simulink library "halin"  (R2021b)
settings: Solver=VariableStepAuto  StartTime=0.0  StopTime=10.0  RelTol=1e-3
undefined symbols (not defined in the file): KHAL_CAN1ABM1E2E_flg, KHAL_CAN1EPB1E2E_flg, KHAL_CAN1EPS1E2E_flg, KHAL_CAN1ESC1E2E_flg, KHAL_CAN1ESC5E2E_flg, KHAL_CAN3BMS1E2E_flg, KHAL_CAN3BMS6E2E_flg, KHAL_CAN3CCU1E2E_flg, KHAL_CAN3CCU2E2E_flg, KHAL_CAN3MCUNF1E2E_flg, KHAL_CAN3MCUNR1E2E_flg, KHAL_CAN3Shifter1E2E_flg, KHAL_CAN3Shifter2E2E_flg, KHAL_CAN6FCM2E2E_flg, KHAL_CAN6FCM4E2E_flg, TRUE
libraries: simulink x645, FVT_lib x212, hcu_lib x59
(part 10 of 23)

== system halin/HAL_IN/CAN2/VHAL_CANMsgInvalidMETER1_flg ==
  Cast To Boolean13 : DataTypeConversion  OutDataTypeStr=boolean
  Constant : Constant  Value=TRUE
  Latch13 : hcu_lib/Basic_Blocks/Latch
  Switch13 : Switch  Criteria=u2 ~= 0
  Unit Delay : UnitDelay  SampleTime=-1  HasFrameUpgradeWarning=on
  UnitConverter : DataTypeConversion  OutDataTypeStr=boolean
  Out : Outport
  wires:
  Constant/1 -> Switch13/3
  Unit Delay/1 -> Cast To Boolean13/1
  Cast To Boolean13/1 -> Switch13/1, Latch13/1
  Switch13/1 -> UnitConverter/1
  Latch13/1 -> Switch13/2
  UnitConverter/1 -> Unit Delay/1, Out/1  "VHAL_CANMsgInvalidMETER1_flg"

== system halin/HAL_IN/CAN3/BMS1 ==
  DT_CAN3_SG_BMS1 : Inport
  0x3C : Constant  Value=0x3C
  0xDC : Constant  Value=0xDC
  BMSChckSum1 : Subsystem
  BMSRolCnct1 : Subsystem
  BitwiseAND{,1..17} (18 alike) : simulink/Logic and Bit Operations/Bitwise Operator  logicop=AND  UseBitMask=on  BitMask=0xFF  BitMaskRealWorld=Stored Integer
  BitwiseOR{,1..6,8..9,11..12,14} (12 alike) : simulink/Logic and Bit Operations/Bitwise Operator  logicop=OR  UseBitMask=off  BitMask=bin2dec('11011001')  BitMaskRealWorld=Stored Integer
  BitwiseOR10 : simulink/Logic and Bit Operations/Bitwise Operator  logicop=OR  UseBitMask=off  NumInputPorts=2  BitMask=bin2dec('11011001')  BitMaskRealWorld=Stored Integer
  BitwiseOR13 : simulink/Logic and Bit Operations/Bitwise Operator  logicop=OR  UseBitMask=off  NumInputPorts=2  BitMask=bin2dec('11011001')  BitMaskRealWorld=Stored Integer
  BitwiseOR7 : simulink/Logic and Bit Operations/Bitwise Operator  logicop=OR  UseBitMask=off  NumInputPorts=2  BitMask=bin2dec('11011001')  BitMaskRealWorld=Stored Integer
  DDM_CS&RC_Comparison : FVT_lib/hal/DDM_CS&RC_Comparison  MsgCycleTime=10
  Data Type Conversion{,1..17} (18 alike) : DataTypeConversion  OutDataTypeStr=uint8
  HVBPwrAvailChrg : Subsystem
  HVBPwrAvailChrg30 : Subsystem
  HVBPwrAvailChrg60 : Subsystem
  HVBPwrAvailDchrg : Subsystem
  HVBPwrAvailDchrg30 : Subsystem
  HVBPwrAvailDchrg60 : Subsystem
  HVBattCurr : Subsystem
  HVBattVolt : Subsystem
  KHAL_CAN3BMS1E2E_flg : Constant  Value=KHAL_CAN3BMS1E2E_flg
  LeftShift : ArithShift  BitShiftDirection=Left
  LeftShift1 : ArithShift  BitShiftDirection=Left
  MessageRollingCounter : FVT_lib/hal/MessageRollingCounter  CounterMAX=14  task_time_ms=5  msg_time_ms=10
  Mux : Mux  Inputs=15
  RightShift{,2,4,12,14} (5 alike) : ArithShift  BitShiftNumber=8
  RightShift{1,3,5,13,15} (5 alike) : ArithShift
  RightShift10 : ArithShift  BitShiftNumber=4
  RightShift11 : ArithShift  BitShiftNumber=-4
  RightShift6 : ArithShift  BitShiftNumber=4
  RightShift7 : ArithShift  BitShiftNumber=-4
  RightShift8 : ArithShift  BitShiftNumber=4
  RightShift9 : ArithShift  BitShiftNumber=-4
  bus_selector : BusSelector  OutputSignals=CAN3_BMSChckSum_1,CAN3_BMSRolCnct_1,CAN3_HVBPwrAvailChrg,CAN3_HVBPwrAvailChrg30,CAN3_HVBPwrAvailChrg60,CAN3_HVBPwrAvailDchrg,CAN3_HVBPwrAvailDchrg30,CAN3_HVBPwrAvailDchrg60,CAN3_HVBattCurr,CAN3_HVBattVolt
  bus_selector1 : BusSelector  OutputSignals=CAN3_BMSChckSum_1
  bus_selector10 : BusSelector  OutputSignals=CAN3_HVBattVolt
  bus_selector2 : BusSelector  OutputSignals=CAN3_BMSRolCnct_1
  bus_selector3 : BusSelector  OutputSignals=CAN3_HVBPwrAvailChrg
  bus_selector4 : BusSelector  OutputSignals=CAN3_HVBPwrAvailChrg30
  bus_selector5 : BusSelector  OutputSignals=CAN3_HVBPwrAvailChrg60
  bus_selector6 : BusSelector  OutputSignals=CAN3_HVBPwrAvailDchrg
  bus_selector7 : BusSelector  OutputSignals=CAN3_HVBPwrAvailDchrg30
  bus_selector8 : BusSelector  OutputSignals=CAN3_HVBPwrAvailDchrg60
  bus_selector9 : BusSelector  OutputSignals=CAN3_HVBattCurr
  constant : Constant  Value=0x0  OutDataTypeStr=uint8
  VHAL_BMS1CSErr_flg : Outport
  VHAL_BMS1RCErr_flg : Outport  Port=2
  VHAL_BMSChckSum1_enum : Outport  Port=3
  VHAL_BMSRolCnct1_enum : Outport  Port=4
  VHAL_HVBPwrAvailChrg_kW : Outport  Port=5
  VHAL_HVBPwrAvailChrg30_kW : Outport  Port=6
  VHAL_HVBPwrAvailChrg60_kW : Outport  Port=7
  VHAL_HVBPwrAvailDchrg_kW : Outport  Port=8
  VHAL_HVBPwrAvailDchrg30_kW : Outport  Port=9
  VHAL_HVBPwrAvailDchrg60_kW : Outport  Port=10
  VHAL_HVBattCurr_A : Outport  Port=11
  VHAL_HVBattVolt_V : Outport  Port=12
  wires:
  DT_CAN3_SG_BMS1/1 -> [DT_CAN3_SG_BMS1]
  [DT_CAN3_SG_BMS1] -> bus_selector/1
  bus_selector/1 -> [CAN3_BMSChckSum_1]  "<CAN3_BMSChckSum_1>"
  [CAN3_BMSChckSum_1] -> LeftShift/1
  LeftShift/1 -> BitwiseAND/1
  BitwiseAND/1 -> [Byte_0_CAN3_BMSChckSum_1]
  bus_selector/2 -> [CAN3_BMSRolCnct_1]  "<CAN3_BMSRolCnct_1>"
  [CAN3_BMSRolCnct_1] -> LeftShift1/1
  LeftShift1/1 -> BitwiseAND1/1
  BitwiseAND1/1 -> [Byte_1_CAN3_BMSRolCnct_1]
  bus_selector/3 -> [CAN3_HVBPwrAvailChrg]  "<CAN3_HVBPwrAvailChrg>"
  [CAN3_HVBPwrAvailChrg] -> RightShift/1, RightShift1/1
  RightShift/1 -> BitwiseAND2/1
  BitwiseAND2/1 -> [Byte_11_CAN3_HVBPwrAvailChrg]
  RightShift1/1 -> BitwiseAND3/1
  BitwiseAND3/1 -> [Byte_12_CAN3_HVBPwrAvailChrg]
  bus_selector/4 -> [CAN3_HVBPwrAvailChrg30]  "<CAN3_HVBPwrAvailChrg30>"
  [CAN3_HVBPwrAvailChrg30] -> RightShift2/1, RightShift3/1
  RightShift2/1 -> BitwiseAND4/1
  BitwiseAND4/1 -> [Byte_14_CAN3_HVBPwrAvailChrg30]
  RightShift3/1 -> BitwiseAND5/1
  BitwiseAND5/1 -> [Byte_15_CAN3_HVBPwrAvailChrg30]
  bus_selector/5 -> [CAN3_HVBPwrAvailChrg60]  "<CAN3_HVBPwrAvailChrg60>"
  [CAN3_HVBPwrAvailChrg60] -> RightShift4/1, RightShift5/1
  RightShift4/1 -> BitwiseAND6/1
  BitwiseAND6/1 -> [Byte_8_CAN3_HVBPwrAvailChrg60]
  RightShift5/1 -> BitwiseAND7/1
  BitwiseAND7/1 -> [Byte_9_CAN3_HVBPwrAvailChrg60]
  bus_selector/6 -> [CAN3_HVBPwrAvailDchrg]  "<CAN3_HVBPwrAvailDchrg>"
  [CAN3_HVBPwrAvailDchrg] -> RightShift6/1, RightShift7/1
  RightShift6/1 -> BitwiseAND8/1
  BitwiseAND8/1 -> [Byte_10_CAN3_HVBPwrAvailDchrg]
  RightShift7/1 -> BitwiseAND9/1
  BitwiseAND9/1 -> [Byte_11_CAN3_HVBPwrAvailDchrg]
  bus_selector/7 -> [CAN3_HVBPwrAvailDchrg30]  "<CAN3_HVBPwrAvailDchrg30>"
  [CAN3_HVBPwrAvailDchrg30] -> RightShift8/1, RightShift9/1
  RightShift8/1 -> BitwiseAND10/1
  BitwiseAND10/1 -> [Byte_13_CAN3_HVBPwrAvailDchrg30]
  RightShift9/1 -> BitwiseAND11/1
  BitwiseAND11/1 -> [Byte_14_CAN3_HVBPwrAvailDchrg30]
  bus_selector/8 -> [CAN3_HVBPwrAvailDchrg60]  "<CAN3_HVBPwrAvailDchrg60>"
  [CAN3_HVBPwrAvailDchrg60] -> RightShift10/1, RightShift11/1
  RightShift10/1 -> BitwiseAND12/1
  BitwiseAND12/1 -> [Byte_7_CAN3_HVBPwrAvailDchrg60]
  RightShift11/1 -> BitwiseAND13/1
  BitwiseAND13/1 -> [Byte_8_CAN3_HVBPwrAvailDchrg60]
  bus_selector/9 -> [CAN3_HVBattCurr]  "<CAN3_HVBattCurr>"
  [CAN3_HVBattCurr] -> RightShift12/1, RightShift13/1
  RightShift12/1 -> BitwiseAND14/1
  BitwiseAND14/1 -> [Byte_5_CAN3_HVBattCurr]
  RightShift13/1 -> BitwiseAND15/1
  BitwiseAND15/1 -> [Byte_6_CAN3_HVBattCurr]
  bus_selector/10 -> [CAN3_HVBattVolt]  "<CAN3_HVBattVolt>"
  [CAN3_HVBattVolt] -> RightShift14/1, RightShift15/1
  RightShift14/1 -> BitwiseAND16/1
  BitwiseAND16/1 -> [Byte_3_CAN3_HVBattVolt]
  RightShift15/1 -> BitwiseAND17/1
  BitwiseAND17/1 -> [Byte_4_CAN3_HVBattVolt]
  Data Type Conversion/1 -> BitwiseOR/1
  [Byte_0_CAN3_BMSChckSum_1] -> Data Type Conversion/1
  BitwiseOR/1 -> [Byte_0]
  Data Type Conversion1/1 -> BitwiseOR1/1
  [Byte_1_CAN3_BMSRolCnct_1] -> Data Type Conversion1/1
  BitwiseOR1/1 -> [Byte_1]
  constant/1 -> [Byte_2]
  Data Type Conversion2/1 -> BitwiseOR2/1
  [Byte_3_CAN3_HVBattVolt] -> Data Type Conversion2/1
  BitwiseOR2/1 -> [Byte_3]
  Data Type Conversion3/1 -> BitwiseOR3/1
  [Byte_4_CAN3_HVBattVolt] -> Data Type Conversion3/1
  BitwiseOR3/1 -> [Byte_4]
  Data Type Conversion4/1 -> BitwiseOR4/1
  [Byte_5_CAN3_HVBattCurr] -> Data Type Conversion4/1
  BitwiseOR4/1 -> [Byte_5]
  Data Type Conversion5/1 -> BitwiseOR5/1
  [Byte_6_CAN3_HVBattCurr] -> Data Type Conversion5/1
  BitwiseOR5/1 -> [Byte_6]
  Data Type Conversion6/1 -> BitwiseOR6/1
  [Byte_7_CAN3_HVBPwrAvailDchrg60] -> Data Type Conversion6/1
  BitwiseOR6/1 -> [Byte_7]
  Data Type Conversion7/1 -> BitwiseOR7/1
  [Byte_8_CAN3_HVBPwrAvailChrg60] -> Data Type Conversion7/1
  Data Type Conversion8/1 -> BitwiseOR7/2
  [Byte_8_CAN3_HVBPwrAvailDchrg60] -> Data Type Conversion8/1
  BitwiseOR7/1 -> [Byte_8]
  Data Type Conversion9/1 -> BitwiseOR8/1
  [Byte_9_CAN3_HVBPwrAvailChrg60] -> Data Type Conversion9/1
  BitwiseOR8/1 -> [Byte_9]
  Data Type Conversion10/1 -> BitwiseOR9/1
  [Byte_10_CAN3_HVBPwrAvailDchrg] -> Data Type Conversion10/1
  BitwiseOR9/1 -> [Byte_10]
  Data Type Conversion11/1 -> BitwiseOR10/1
  [Byte_11_CAN3_HVBPwrAvailChrg] -> Data Type Conversion11/1
  Data Type Conversion12/1 -> BitwiseOR10/2
  [Byte_11_CAN3_HVBPwrAvailDchrg] -> Data Type Conversion12/1
  BitwiseOR10/1 -> [Byte_11]
  Data Type Conversion13/1 -> BitwiseOR11/1
  [Byte_12_CAN3_HVBPwrAvailChrg] -> Data Type Conversion13/1
  BitwiseOR11/1 -> [Byte_12]
  Data Type Conversion14/1 -> BitwiseOR12/1
  [Byte_13_CAN3_HVBPwrAvailDchrg30] -> Data Type Conversion14/1
  BitwiseOR12/1 -> [Byte_13]
  Data Type Conversion15/1 -> BitwiseOR13/1
  [Byte_14_CAN3_HVBPwrAvailChrg30] -> Data Type Conversion15/1
  Data Type Conversion16/1 -> BitwiseOR13/2
  [Byte_14_CAN3_HVBPwrAvailDchrg30] -> Data Type Conversion16/1
  BitwiseOR13/1 -> [Byte_14]
  Data Type Conversion17/1 -> BitwiseOR14/1
  [Byte_15_CAN3_HVBPwrAvailChrg30] -> Data Type Conversion17/1
  BitwiseOR14/1 -> [Byte_15]
  [Byte_1] -> Mux/1
  [Byte_2] -> Mux/2
  [Byte_3] -> Mux/3
  [Byte_4] -> Mux/4
  [Byte_5] -> Mux/5
  [Byte_6] -> Mux/6
  [Byte_7] -> Mux/7
  [Byte_8] -> Mux/8
  [Byte_9] -> Mux/9
  [Byte_10] -> Mux/10
  [Byte_11] -> Mux/11
  [Byte_12] -> Mux/12
  [Byte_13] -> Mux/13
  [Byte_14] -> Mux/14
  [Byte_15] -> Mux/15
  Mux/1 -> [VHAL_CAN3BMS1noCS_raw]
  KHAL_CAN3BMS1E2E_flg/1 -> DDM_CS&RC_Comparison/1
  0x3C/1 -> DDM_CS&RC_Comparison/2
  0xDC/1 -> DDM_CS&RC_Comparison/3
  [VHAL_CAN3BMS1noCS_raw] -> DDM_CS&RC_Comparison/4
  [Byte_0] -> DDM_CS&RC_Comparison/5
  [RC_ECU] -> DDM_CS&RC_Comparison/6
  MessageRollingCounter/1 -> DDM_CS&RC_Comparison/7
  DDM_CS&RC_Comparison/1 -> VHAL_BMS1CSErr_flg/1
  DDM_CS&RC_Comparison/2 -> VHAL_BMS1RCErr_flg/1
  [DT_CAN3_SG_BMS1] -> bus_selector1/1
  bus_selector1/1 -> BMSChckSum1/1(BMSChckSum_1)  "<CAN3_BMSChckSum_1>"
  BMSChckSum1/1(VHAL_BMSChckSum1_enum) -> VHAL_BMSChckSum1_enum/1
  [DT_CAN3_SG_BMS1] -> bus_selector2/1
  bus_selector2/1 -> BMSRolCnct1/1(BMSRolCnct_1)  "<CAN3_BMSRolCnct_1>"
  BMSRolCnct1/1(VHAL_BMSRolCnct1_enum) -> VHAL_BMSRolCnct1_enum/1, [RC_ECU]
  [DT_CAN3_SG_BMS1] -> bus_selector3/1
  bus_selector3/1 -> HVBPwrAvailChrg/1(HVBPwrAvailChrg)  "<CAN3_HVBPwrAvailChrg>"
  HVBPwrAvailChrg/1(VHAL_HVBPwrAvailChrg_kW) -> VHAL_HVBPwrAvailChrg_kW/1
  [DT_CAN3_SG_BMS1] -> bus_selector4/1
  bus_selector4/1 -> HVBPwrAvailChrg30/1(HVBPwrAvailChrg30)  "<CAN3_HVBPwrAvailChrg30>"
  HVBPwrAvailChrg30/1(VHAL_HVBPwrAvailChrg30_kW) -> VHAL_HVBPwrAvailChrg30_kW/1
  [DT_CAN3_SG_BMS1] -> bus_selector5/1
  bus_selector5/1 -> HVBPwrAvailChrg60/1(HVBPwrAvailChrg60)  "<CAN3_HVBPwrAvailChrg60>"
  HVBPwrAvailChrg60/1(VHAL_HVBPwrAvailChrg60_kW) -> VHAL_HVBPwrAvailChrg60_kW/1
  [DT_CAN3_SG_BMS1] -> bus_selector6/1
  bus_selector6/1 -> HVBPwrAvailDchrg/1(HVBPwrAvailDchrg)  "<CAN3_HVBPwrAvailDchrg>"
  HVBPwrAvailDchrg/1(VHAL_HVBPwrAvailDchrg_kW) -> VHAL_HVBPwrAvailDchrg_kW/1
  [DT_CAN3_SG_BMS1] -> bus_selector7/1
  bus_selector7/1 -> HVBPwrAvailDchrg30/1(HVBPwrAvailDchrg30)  "<CAN3_HVBPwrAvailDchrg30>"
  HVBPwrAvailDchrg30/1(VHAL_HVBPwrAvailDchrg30_kW) -> VHAL_HVBPwrAvailDchrg30_kW/1
  [DT_CAN3_SG_BMS1] -> bus_selector8/1
  bus_selector8/1 -> HVBPwrAvailDchrg60/1(HVBPwrAvailDchrg60)  "<CAN3_HVBPwrAvailDchrg60>"
  HVBPwrAvailDchrg60/1(VHAL_HVBPwrAvailDchrg60_kW) -> VHAL_HVBPwrAvailDchrg60_kW/1
  [DT_CAN3_SG_BMS1] -> bus_selector9/1
  bus_selector9/1 -> HVBattCurr/1(HVBattCurr)  "<CAN3_HVBattCurr>"
  HVBattCurr/1(VHAL_HVBattCurr_A) -> VHAL_HVBattCurr_A/1
  [DT_CAN3_SG_BMS1] -> bus_selector10/1
  bus_selector10/1 -> HVBattVolt/1(HVBattVolt)  "<CAN3_HVBattVolt>"
  HVBattVolt/1(VHAL_HVBattVolt_V) -> VHAL_HVBattVolt_V/1

== system halin/HAL_IN/CAN3/BMS3 ==
  DT_CAN3_SG_BMS3 : Inport
  ACChrgCurrDis : Subsystem
  FireDetErr : Subsystem
  HVBChrgPwr : Subsystem
  HVBChrgPwrTotal : Subsystem
  HVBDrvPwr : Subsystem
  HVBDrvPwrTotal : Subsystem
  HVBFullChrgPwr : Subsystem
  HVBIsoImpedenceN : Subsystem
  HVBIsoImpedenceP : Subsystem
  HVBSOH : Subsystem
  HVBattErr : Subsystem
  HVBattPackVolt : Subsystem
  HVBattSOC : Subsystem
  HVBattSOCDis : Subsystem
  RemainChrgTime : Subsystem
  bus_selector : BusSelector  OutputSignals=CAN3_ACChrgCurrDis
  bus_selector1 : BusSelector  OutputSignals=CAN3_FireDetErr
  bus_selector10 : BusSelector  OutputSignals=CAN3_HVBattErr
  bus_selector11 : BusSelector  OutputSignals=CAN3_HVBattPackVolt
  bus_selector12 : BusSelector  OutputSignals=CAN3_HVBattSOC
  bus_selector13 : BusSelector  OutputSignals=CAN3_HVBattSOCDis
  bus_selector14 : BusSelector  OutputSignals=CAN3_RemainChrgTime
  bus_selector2 : BusSelector  OutputSignals=CAN3_HVBChrgPwr
  bus_selector3 : BusSelector  OutputSignals=CAN3_HVBChrgPwrTotal
  bus_selector4 : BusSelector  OutputSignals=CAN3_HVBDrvPwr
  bus_selector5 : BusSelector  OutputSignals=CAN3_HVBDrvPwrTotal
  bus_selector6 : BusSelector  OutputSignals=CAN3_HVBFullChrgPwr
  bus_selector7 : BusSelector  OutputSignals=CAN3_HVBIsoImpedenceN
  bus_selector8 : BusSelector  OutputSignals=CAN3_HVBIsoImpedenceP
  bus_selector9 : BusSelector  OutputSignals=CAN3_HVBSOH
  VHAL_ACChrgCurrDis_A : Outport
  VHAL_FireDetErr_flg : Outport  Port=2
  VHAL_HVBChrgPwr_kWh : Outport  Port=3
  VHAL_HVBChrgPwrTotal_kWh : Outport  Port=4
  VHAL_HVBDrvPwr_kWh : Outport  Port=5
  VHAL_HVBDrvPwrTotal_kWh : Outport  Port=6
  VHAL_HVBFullChrgPwr_kWh : Outport  Port=7
  VHAL_HVBIsoImpedenceN_Megaohm : Outport  Port=8
  VHAL_HVBIsoImpedenceP_Megaohm : Outport  Port=9
  VHAL_HVBSOH_pct : Outport  Port=10
  VHAL_HVBattErr_flg : Outport  Port=11
  VHAL_HVBattPackVolt_V : Outport  Port=12
  VHAL_HVBattSOC_pct : Outport  Port=13
  VHAL_HVBattSOCDis_pct : Outport  Port=14
  VHAL_RemainChrgTime_min : Outport  Port=15
  wires:
  DT_CAN3_SG_BMS3/1 -> [DT_CAN3_SG_BMS3]
  [DT_CAN3_SG_BMS3] -> bus_selector/1
  bus_selector/1 -> ACChrgCurrDis/1(ACChrgCurrDis)  "<CAN3_ACChrgCurrDis>"
  ACChrgCurrDis/1(VHAL_ACChrgCurrDis_A) -> VHAL_ACChrgCurrDis_A/1
  [DT_CAN3_SG_BMS3] -> bus_selector1/1
  bus_selector1/1 -> FireDetErr/1(FireDetErr)  "<CAN3_FireDetErr>"
  FireDetErr/1(VHAL_FireDetErr_flg) -> VHAL_FireDetErr_flg/1
  [DT_CAN3_SG_BMS3] -> bus_selector2/1
  bus_selector2/1 -> HVBChrgPwr/1(HVBChrgPwr)  "<CAN3_HVBChrgPwr>"
  HVBChrgPwr/1(VHAL_HVBChrgPwr_kWh) -> VHAL_HVBChrgPwr_kWh/1
  [DT_CAN3_SG_BMS3] -> bus_selector3/1
  bus_selector3/1 -> HVBChrgPwrTotal/1(HVBChrgPwrTotal)  "<CAN3_HVBChrgPwrTotal>"
  HVBChrgPwrTotal/1(VHAL_HVBChrgPwrTotal_kWh) -> VHAL_HVBChrgPwrTotal_kWh/1
  [DT_CAN3_SG_BMS3] -> bus_selector4/1
  bus_selector4/1 -> HVBDrvPwr/1(HVBDrvPwr)  "<CAN3_HVBDrvPwr>"
  HVBDrvPwr/1(VHAL_HVBDrvPwr_kWh) -> VHAL_HVBDrvPwr_kWh/1
  [DT_CAN3_SG_BMS3] -> bus_selector5/1
  bus_selector5/1 -> HVBDrvPwrTotal/1(HVBDrvPwrTotal)  "<CAN3_HVBDrvPwrTotal>"
  HVBDrvPwrTotal/1(VHAL_HVBDrvPwrTotal_kWh) -> VHAL_HVBDrvPwrTotal_kWh/1
  [DT_CAN3_SG_BMS3] -> bus_selector6/1
  bus_selector6/1 -> HVBFullChrgPwr/1(HVBFullChrgPwr)  "<CAN3_HVBFullChrgPwr>"
  HVBFullChrgPwr/1(VHAL_HVBFullChrgPwr_kWh) -> VHAL_HVBFullChrgPwr_kWh/1
  [DT_CAN3_SG_BMS3] -> bus_selector7/1
  bus_selector7/1 -> HVBIsoImpedenceN/1(HVBIsoImpedenceN)  "<CAN3_HVBIsoImpedenceN>"
  HVBIsoImpedenceN/1(VHAL_HVBIsoImpedenceN_Megaohm) -> VHAL_HVBIsoImpedenceN_Megaohm/1
  [DT_CAN3_SG_BMS3] -> bus_selector8/1
  bus_selector8/1 -> HVBIsoImpedenceP/1(HVBIsoImpedenceP)  "<CAN3_HVBIsoImpedenceP>"
  HVBIsoImpedenceP/1(VHAL_HVBIsoImpedenceP_Megaohm) -> VHAL_HVBIsoImpedenceP_Megaohm/1
  [DT_CAN3_SG_BMS3] -> bus_selector9/1
  bus_selector9/1 -> HVBSOH/1(HVBSOH)  "<CAN3_HVBSOH>"
  HVBSOH/1(VHAL_HVBSOH_pct) -> VHAL_HVBSOH_pct/1
  [DT_CAN3_SG_BMS3] -> bus_selector10/1
  bus_selector10/1 -> HVBattErr/1(HVBattErr)  "<CAN3_HVBattErr>"
  HVBattErr/1(VHAL_HVBattErr_flg) -> VHAL_HVBattErr_flg/1
  [DT_CAN3_SG_BMS3] -> bus_selector11/1
  bus_selector11/1 -> HVBattPackVolt/1(HVBattPackVolt)  "<CAN3_HVBattPackVolt>"
  HVBattPackVolt/1(VHAL_HVBattPackVolt_V) -> VHAL_HVBattPackVolt_V/1
  [DT_CAN3_SG_BMS3] -> bus_selector12/1
  bus_selector12/1 -> HVBattSOC/1(HVBattSOC)  "<CAN3_HVBattSOC>"
  HVBattSOC/1(VHAL_HVBattSOC_pct) -> VHAL_HVBattSOC_pct/1
  [DT_CAN3_SG_BMS3] -> bus_selector13/1
  bus_selector13/1 -> HVBattSOCDis/1(HVBattSOCDis)  "<CAN3_HVBattSOCDis>"
  HVBattSOCDis/1(VHAL_HVBattSOCDis_pct) -> VHAL_HVBattSOCDis_pct/1
  [DT_CAN3_SG_BMS3] -> bus_selector14/1
  bus_selector14/1 -> RemainChrgTime/1(RemainChrgTime)  "<CAN3_RemainChrgTime>"
  RemainChrgTime/1(VHAL_RemainChrgTime_min) -> VHAL_RemainChrgTime_min/1

== system halin/HAL_IN/CAN3/BMS4 ==
  DT_CAN3_SG_BMS4 : Inport
  CellTempAvg : Subsystem
  HVBCellVoltMax : Subsystem
  HVBCellVoltMin : Subsystem
  HVBMTempMax : Subsystem
  HVBMTempMin : Subsystem
  MaxCellTempNum : Subsystem
  MaxCellVoltNum : Subsystem
  MinCellTempNum : Subsystem
  MinCellVoltNum : Subsystem
  bus_selector : BusSelector  OutputSignals=CAN3_CellTempAvg
  bus_selector1 : BusSelector  OutputSignals=CAN3_HVBCellVoltMax
  bus_selector2 : BusSelector  OutputSignals=CAN3_HVBCellVoltMin
  bus_selector3 : BusSelector  OutputSignals=CAN3_HVBMTempMax
  bus_selector4 : BusSelector  OutputSignals=CAN3_HVBMTempMin
  bus_selector5 : BusSelector  OutputSignals=CAN3_MaxCellTemp_Num
  bus_selector6 : BusSelector  OutputSignals=CAN3_MaxCellVolt_Num
  bus_selector7 : BusSelector  OutputSignals=CAN3_MinCellTemp_Num
  bus_selector8 : BusSelector  OutputSignals=CAN3_MinCellVolt_Num
  VHAL_CellTempAvg_C : Outport
  VHAL_HVBCellVoltMax_mV : Outport  Port=2
  VHAL_HVBCellVoltMin_mV : Outport  Port=3
  VHAL_HVBMTempMax_C : Outport  Port=4
  VHAL_HVBMTempMin_C : Outport  Port=5
  VHAL_MaxCellTempNum_enum : Outport  Port=6
  VHAL_MaxCellVoltNum_enum : Outport  Port=7
  VHAL_MinCellTempNum_enum : Outport  Port=8
  VHAL_MinCellVoltNum_enum : Outport  Port=9
  wires:
  DT_CAN3_SG_BMS4/1 -> [DT_CAN3_SG_BMS4]
  [DT_CAN3_SG_BMS4] -> bus_selector/1
  bus_selector/1 -> CellTempAvg/1(CellTempAvg)  "<CAN3_CellTempAvg>"
  CellTempAvg/1(VHAL_CellTempAvg_C) -> VHAL_CellTempAvg_C/1
  [DT_CAN3_SG_BMS4] -> bus_selector1/1
  bus_selector1/1 -> HVBCellVoltMax/1(HVBCellVoltMax)  "<CAN3_HVBCellVoltMax>"
  HVBCellVoltMax/1(VHAL_HVBCellVoltMax_mV) -> VHAL_HVBCellVoltMax_mV/1
  [DT_CAN3_SG_BMS4] -> bus_selector2/1
  bus_selector2/1 -> HVBCellVoltMin/1(HVBCellVoltMin)  "<CAN3_HVBCellVoltMin>"
  HVBCellVoltMin/1(VHAL_HVBCellVoltMin_mV) -> VHAL_HVBCellVoltMin_mV/1
  [DT_CAN3_SG_BMS4] -> bus_selector3/1
  bus_selector3/1 -> HVBMTempMax/1(HVBMTempMax)  "<CAN3_HVBMTempMax>"
  HVBMTempMax/1(VHAL_HVBMTempMax_C) -> VHAL_HVBMTempMax_C/1
  [DT_CAN3_SG_BMS4] -> bus_selector4/1
  bus_selector4/1 -> HVBMTempMin/1(HVBMTempMin)  "<CAN3_HVBMTempMin>"
  HVBMTempMin/1(VHAL_HVBMTempMin_C) -> VHAL_HVBMTempMin_C/1
  [DT_CAN3_SG_BMS4] -> bus_selector5/1
  bus_selector5/1 -> MaxCellTempNum/1(MaxCellTemp_Num)  "<CAN3_MaxCellTemp_Num>"
  MaxCellTempNum/1(VHAL_MaxCellTempNum_enum) -> VHAL_MaxCellTempNum_enum/1
  [DT_CAN3_SG_BMS4] -> bus_selector6/1
  bus_selector6/1 -> MaxCellVoltNum/1(MaxCellVolt_Num)  "<CAN3_MaxCellVolt_Num>"
  MaxCellVoltNum/1(VHAL_MaxCellVoltNum_enum) -> VHAL_MaxCellVoltNum_enum/1
  [DT_CAN3_SG_BMS4] -> bus_selector7/1
  bus_selector7/1 -> MinCellTempNum/1(MinCellTemp_Num)  "<CAN3_MinCellTemp_Num>"
  MinCellTempNum/1(VHAL_MinCellTempNum_enum) -> VHAL_MinCellTempNum_enum/1
  [DT_CAN3_SG_BMS4] -> bus_selector8/1
  bus_selector8/1 -> MinCellVoltNum/1(MinCellVolt_Num)  "<CAN3_MinCellVolt_Num>"
  MinCellVoltNum/1(VHAL_MinCellVoltNum_enum) -> VHAL_MinCellVoltNum_enum/1

== system halin/HAL_IN/CAN3/BMS5 ==
  DT_CAN3_SG_BMS5 : Inport
  HVInVolt : Subsystem
  LVBattDet12V : Subsystem
  OBCACCSLimit : Subsystem
  OBCDCCurLm : Subsystem
  OBCDCVoltLm : Subsystem
  bus_selector : BusSelector  OutputSignals=CAN3_HVInVolt
  bus_selector1 : BusSelector  OutputSignals=CAN3_LVBattDet12V
  bus_selector2 : BusSelector  OutputSignals=CAN3_OBCACCSLimit
  bus_selector3 : BusSelector  OutputSignals=CAN3_OBCDCCurLm
  bus_selector4 : BusSelector  OutputSignals=CAN3_OBCDCVoltLm
  VHAL_HVInVolt_V : Outport
  VHAL_LVBattDet12V_V : Outport  Port=2
  VHAL_OBCACCSLimit_A : Outport  Port=3
  VHAL_OBCDCCurLm_A : Outport  Port=4
  VHAL_OBCDCVoltLm_V : Outport  Port=5
  wires:
  DT_CAN3_SG_BMS5/1 -> [DT_CAN3_SG_BMS5]
  [DT_CAN3_SG_BMS5] -> bus_selector/1
  bus_selector/1 -> HVInVolt/1(HVInVolt)  "<CAN3_HVInVolt>"
  HVInVolt/1(VHAL_HVInVolt_V) -> VHAL_HVInVolt_V/1
  [DT_CAN3_SG_BMS5] -> bus_selector1/1
  bus_selector1/1 -> LVBattDet12V/1(LVBattDet12V)  "<CAN3_LVBattDet12V>"
  LVBattDet12V/1(VHAL_LVBattDet12V_V) -> VHAL_LVBattDet12V_V/1
  [DT_CAN3_SG_BMS5] -> bus_selector2/1
  bus_selector2/1 -> OBCACCSLimit/1(OBCACCSLimit)  "<CAN3_OBCACCSLimit>"
  OBCACCSLimit/1(VHAL_OBCACCSLimit_A) -> VHAL_OBCACCSLimit_A/1
  [DT_CAN3_SG_BMS5] -> bus_selector3/1
  bus_selector3/1 -> OBCDCCurLm/1(OBCDCCurLm)  "<CAN3_OBCDCCurLm>"
  OBCDCCurLm/1(VHAL_OBCDCCurLm_A) -> VHAL_OBCDCCurLm_A/1
  [DT_CAN3_SG_BMS5] -> bus_selector4/1
  bus_selector4/1 -> OBCDCVoltLm/1(OBCDCVoltLm)  "<CAN3_OBCDCVoltLm>"
  OBCDCVoltLm/1(VHAL_OBCDCVoltLm_V) -> VHAL_OBCDCVoltLm_V/1

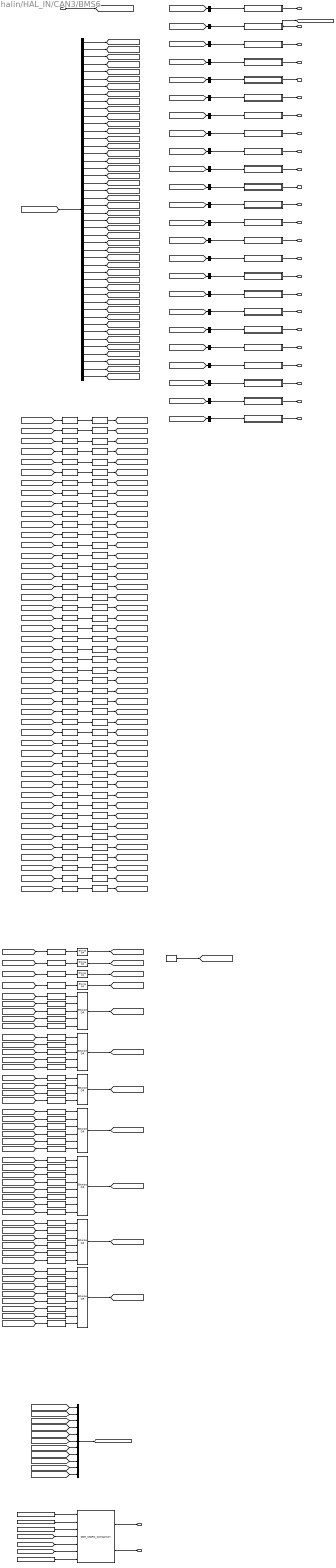
== system halin/HAL_IN/CAN3/BMS6 ==
  DT_CAN3_SG_BMS6 : Inport
  0x3B : Constant  Value=0x3B
  0xDB : Constant  Value=0xDB
  BMSChckSum : Subsystem
  BMSREADY : Subsystem
  BMSRolCnct : Subsystem
  BMSWarn1 : Subsystem
  BMSWarn2 : Subsystem
  BMSWarn3 : Subsystem
  BMSWarn4 : Subsystem
  BMSWarn5 : Subsystem
  BMSWarn6 : Subsystem
  BMSWarn7 : Subsystem
  BMSWarn8 : Subsystem
  BitwiseAND{,1..45} (46 alike) : simulink/Logic and Bit Operations/Bitwise Operator  logicop=AND  UseBitMask=on  BitMask=0xFF  BitMaskRealWorld=Stored Integer
  BitwiseOR{,1..3} (4 alike) : simulink/Logic and Bit Operations/Bitwise Operator  logicop=OR  UseBitMask=off  BitMask=bin2dec('11011001')  BitMaskRealWorld=Stored Integer
  BitwiseOR10 : simulink/Logic and Bit Operations/Bitwise Operator  logicop=OR  UseBitMask=off  NumInputPorts=8  BitMask=bin2dec('11011001')  BitMaskRealWorld=Stored Integer
  BitwiseOR4 : simulink/Logic and Bit Operations/Bitwise Operator  logicop=OR  UseBitMask=off  NumInputPorts=5  BitMask=bin2dec('11011001')  BitMaskRealWorld=Stored Integer
  BitwiseOR5 : simulink/Logic and Bit Operations/Bitwise Operator  logicop=OR  UseBitMask=off  NumInputPorts=5  BitMask=bin2dec('11011001')  BitMaskRealWorld=Stored Integer
  BitwiseOR6 : simulink/Logic and Bit Operations/Bitwise Operator  logicop=OR  UseBitMask=off  NumInputPorts=4  BitMask=bin2dec('11011001')  BitMaskRealWorld=Stored Integer
  BitwiseOR7 : simulink/Logic and Bit Operations/Bitwise Operator  logicop=OR  UseBitMask=off  NumInputPorts=6  BitMask=bin2dec('11011001')  BitMaskRealWorld=Stored Integer
  BitwiseOR8 : simulink/Logic and Bit Operations/Bitwise Operator  logicop=OR  UseBitMask=off  NumInputPorts=8  BitMask=bin2dec('11011001')  BitMaskRealWorld=Stored Integer
  BitwiseOR9 : simulink/Logic and Bit Operations/Bitwise Operator  logicop=OR  UseBitMask=off  NumInputPorts=6  BitMask=bin2dec('11011001')  BitMaskRealWorld=Stored Integer
  ChrgInLockReq : Subsystem
  ChrgPlugSta : Subsystem
  DDM_CS&RC_Comparison : FVT_lib/hal/DDM_CS&RC_Comparison  MsgCycleTime=100
  Data Type Conversion{,1..45} (46 alike) : DataTypeConversion  OutDataTypeStr=uint8
  DisChrgPlugErr : Subsystem
  ExtChrgSta : Subsystem
  HVBChrgErr : Subsystem
  HVBContactorSta : Subsystem
  HVBHVILErr : Subsystem
  HVBOvrTempErr : Subsystem
  HVBOvrTempWarn : Subsystem
  HVBPreheatPrecoolSta : Subsystem
  HVBattReady4Pre : Subsystem
  HVILSta : Subsystem
  KHAL_CAN3BMS6E2E_flg : Constant  Value=KHAL_CAN3BMS6E2E_flg
  LeftShift{,1,3,14,17,22,25,29,41,43,45} (11 alike) : ArithShift  BitShiftDirection=Left
  LeftShift{10,24,35,42} (4 alike) : ArithShift  BitShiftNumber=7  BitShiftDirection=Left
  LeftShift{5,11,13,20,23,28,39} (7 alike) : ArithShift  BitShiftNumber=2  BitShiftDirection=Left
  LeftShift{7,12,16,18,27,30..31} (7 alike) : ArithShift  BitShiftNumber=4  BitShiftDirection=Left
  LeftShift{9,15,19,32..34,36} (7 alike) : ArithShift  BitShiftNumber=6  BitShiftDirection=Left
  LeftShift{2,4,21,26,44} (5 alike) : ArithShift  BitShiftNumber=1  BitShiftDirection=Left
  LeftShift37 : ArithShift  BitShiftNumber=5  BitShiftDirection=Left
  LeftShift38 : ArithShift  BitShiftNumber=3  BitShiftDirection=Left
  LeftShift40 : ArithShift  BitShiftNumber=5  BitShiftDirection=Left
  LeftShift6 : ArithShift  BitShiftNumber=3  BitShiftDirection=Left
  LeftShift8 : ArithShift  BitShiftNumber=5  BitShiftDirection=Left
  MessageRollingCounter : FVT_lib/hal/MessageRollingCounter  CounterMAX=14  task_time_ms=5  msg_time_ms=100
  Mux : Mux  Inputs=11
  V2LSta : Subsystem
  bus_selector : BusSelector  OutputSignals=CAN3_BMSChckSum,CAN3_BMSRolCnct,CAN3_BMS_READY,CAN3_BMS_Warn_1,CAN3_BMS_Warn_2,CAN3_BMS_Warn_3,CAN3_BMS_Warn_4,CAN3_BMS_Warn_5,CAN3_BMS_Warn_6,CAN3_BMS_Warn_7,CAN3_BMS_Warn_8,CAN3_CellUnconsistErr,CAN3_ChrgInLockReq,CAN3_ChrgPlugSta,CAN3_DCChrgSysShockErr,CAN3_DisChrgPlugErr,CAN3_ExtChrgSta,CAN3_HVBCellOvrVoltErr,CAN3_HVBCellOvrVoltWarn,CAN3_HVBCellUdrVoltWarn,CAN3_HVBCellUnbalanErr,CAN3_HVBCellUndrVoltErr,CAN3_HVBChrgErr,CAN3_HVBContactorSta,CAN3_HVBHVILErr,CAN3_HVBOvrChrgCurrErr,CAN3_HVBOvrDchrgCurErr,CAN3_HVBOvrSOCErr,CAN3_HVBOvrTempErr,CAN3_HVBOvrTempWarn,CAN3_HVBOvrVoltErr,CAN3_HVBPrechrgSta,CAN3_HVBPreheatPrecoolSta,CAN3_HVBSOCJumpError,CAN3_HVBShrtChrgCurrErr,CAN3_HVBShrtDischrgCurrErr,CAN3_HVBTempDiffErr,CAN3_HVBUndrSOCErr,CAN3_HVBUndrTempErr,CAN3_HVBUndrTempWarn,CAN3_HVBUndrVoltErr,CAN3_HVBattReady4Pre,CAN3_HVILSta,CAN3_IsoDetSta,CAN3_SystemUncomErr,CAN3_V2LSta
  bus_selector1 : BusSelector  OutputSignals=CAN3_BMSChckSum
  bus_selector10 : BusSelector  OutputSignals=CAN3_BMS_Warn_7
  bus_selector11 : BusSelector  OutputSignals=CAN3_BMS_Warn_8
  bus_selector12 : BusSelector  OutputSignals=CAN3_ChrgInLockReq
  bus_selector13 : BusSelector  OutputSignals=CAN3_ChrgPlugSta
  bus_selector14 : BusSelector  OutputSignals=CAN3_DisChrgPlugErr
  bus_selector15 : BusSelector  OutputSignals=CAN3_ExtChrgSta
  bus_selector16 : BusSelector  OutputSignals=CAN3_HVBChrgErr
  bus_selector17 : BusSelector  OutputSignals=CAN3_HVBContactorSta
  bus_selector18 : BusSelector  OutputSignals=CAN3_HVBHVILErr
  bus_selector19 : BusSelector  OutputSignals=CAN3_HVBOvrTempErr
  bus_selector2 : BusSelector  OutputSignals=CAN3_BMSRolCnct
  bus_selector20 : BusSelector  OutputSignals=CAN3_HVBOvrTempWarn
  bus_selector21 : BusSelector  OutputSignals=CAN3_HVBPreheatPrecoolSta
  bus_selector22 : BusSelector  OutputSignals=CAN3_HVBattReady4Pre
  bus_selector23 : BusSelector  OutputSignals=CAN3_HVILSta
  bus_selector24 : BusSelector  OutputSignals=CAN3_V2LSta
  bus_selector3 : BusSelector  OutputSignals=CAN3_BMS_READY
  bus_selector4 : BusSelector  OutputSignals=CAN3_BMS_Warn_1
  bus_selector5 : BusSelector  OutputSignals=CAN3_BMS_Warn_2
  bus_selector6 : BusSelector  OutputSignals=CAN3_BMS_Warn_3
  bus_selector7 : BusSelector  OutputSignals=CAN3_BMS_Warn_4
  bus_selector8 : BusSelector  OutputSignals=CAN3_BMS_Warn_5
  bus_selector9 : BusSelector  OutputSignals=CAN3_BMS_Warn_6
  constant : Constant  Value=0x0  OutDataTypeStr=uint8
  VHAL_BMS6CSErr_flg : Outport
  VHAL_BMS6RCErr_flg : Outport  Port=2
  VHAL_BMSChckSum_enum : Outport  Port=3
  VHAL_BMSRolCnct_enum : Outport  Port=4
  VHAL_BMSREADY_flg : Outport  Port=5
  VHAL_BMSWarn1_flg : Outport  Port=6
  VHAL_BMSWarn2_flg : Outport  Port=7
  VHAL_BMSWarn3_flg : Outport  Port=8
  VHAL_BMSWarn4_flg : Outport  Port=9
  VHAL_BMSWarn5_flg : Outport  Port=10
  VHAL_BMSWarn6_flg : Outport  Port=11
  VHAL_BMSWarn7_flg : Outport  Port=12
  VHAL_BMSWarn8_flg : Outport  Port=13
  VHAL_ChrgInLockReq_enum : Outport  Port=14
  VHAL_ChrgPlugSta_enum : Outport  Port=15
  VHAL_DisChrgPlugErr_enum : Outport  Port=16
  VHAL_ExtChrgSta_enum : Outport  Port=17
  VHAL_HVBChrgErr_enum : Outport  Port=18
  VHAL_HVBContactorSta_flg : Outport  Port=19
  VHAL_HVBHVILErr_flg : Outport  Port=20
  VHAL_HVBOvrTempErr_flg : Outport  Port=21
  VHAL_HVBOvrTempWarn_enum : Outport  Port=22
  VHAL_HVBPreheatPrecoolSta_enum : Outport  Port=23
  VHAL_HVBattReady4Pre_enum : Outport  Port=24
  VHAL_HVILSta_flg : Outport  Port=25
  VHAL_V2LSta_enum : Outport  Port=26
  wires:
  DT_CAN3_SG_BMS6/1 -> [DT_CAN3_SG_BMS6]
  [DT_CAN3_SG_BMS6] -> bus_selector/1
  bus_selector/1 -> [CAN3_BMSChckSum]  "<CAN3_BMSChckSum>"
  [CAN3_BMSChckSum] -> LeftShift/1
  LeftShift/1 -> BitwiseAND/1
  BitwiseAND/1 -> [Byte_0_CAN3_BMSChckSum]
  bus_selector/2 -> [CAN3_BMSRolCnct]  "<CAN3_BMSRolCnct>"
  [CAN3_BMSRolCnct] -> LeftShift1/1
  LeftShift1/1 -> BitwiseAND1/1
  BitwiseAND1/1 -> [Byte_1_CAN3_BMSRolCnct]
  bus_selector/3 -> [CAN3_BMS_READY]  "<CAN3_BMS_READY>"
  [CAN3_BMS_READY] -> LeftShift2/1
  LeftShift2/1 -> BitwiseAND2/1
  BitwiseAND2/1 -> [Byte_8_CAN3_BMS_READY]
  bus_selector/4 -> [CAN3_BMS_Warn_1]  "<CAN3_BMS_Warn_1>"
  [CAN3_BMS_Warn_1] -> LeftShift3/1
  LeftShift3/1 -> BitwiseAND3/1
  BitwiseAND3/1 -> [Byte_11_CAN3_BMS_Warn_1]
  bus_selector/5 -> [CAN3_BMS_Warn_2]  "<CAN3_BMS_Warn_2>"
  [CAN3_BMS_Warn_2] -> LeftShift4/1
  LeftShift4/1 -> BitwiseAND4/1
  BitwiseAND4/1 -> [Byte_11_CAN3_BMS_Warn_2]
  bus_selector/6 -> [CAN3_BMS_Warn_3]  "<CAN3_BMS_Warn_3>"
  [CAN3_BMS_Warn_3] -> LeftShift5/1
  LeftShift5/1 -> BitwiseAND5/1
  BitwiseAND5/1 -> [Byte_11_CAN3_BMS_Warn_3]
  bus_selector/7 -> [CAN3_BMS_Warn_4]  "<CAN3_BMS_Warn_4>"
  [CAN3_BMS_Warn_4] -> LeftShift6/1
  LeftShift6/1 -> BitwiseAND6/1
  BitwiseAND6/1 -> [Byte_11_CAN3_BMS_Warn_4]
  bus_selector/8 -> [CAN3_BMS_Warn_5]  "<CAN3_BMS_Warn_5>"
  [CAN3_BMS_Warn_5] -> LeftShift7/1
  LeftShift7/1 -> BitwiseAND7/1
  BitwiseAND7/1 -> [Byte_11_CAN3_BMS_Warn_5]
  bus_selector/9 -> [CAN3_BMS_Warn_6]  "<CAN3_BMS_Warn_6>"
  [CAN3_BMS_Warn_6] -> LeftShift8/1
  LeftShift8/1 -> BitwiseAND8/1
  BitwiseAND8/1 -> [Byte_11_CAN3_BMS_Warn_6]
  bus_selector/10 -> [CAN3_BMS_Warn_7]  "<CAN3_BMS_Warn_7>"
  [CAN3_BMS_Warn_7] -> LeftShift9/1
  LeftShift9/1 -> BitwiseAND9/1
  BitwiseAND9/1 -> [Byte_11_CAN3_BMS_Warn_7]
  bus_selector/11 -> [CAN3_BMS_Warn_8]  "<CAN3_BMS_Warn_8>"
  [CAN3_BMS_Warn_8] -> LeftShift10/1
  LeftShift10/1 -> BitwiseAND10/1
  BitwiseAND10/1 -> [Byte_11_CAN3_BMS_Warn_8]
  bus_selector/12 -> [CAN3_CellUnconsistErr]  "<CAN3_CellUnconsistErr>"
  [CAN3_CellUnconsistErr] -> LeftShift11/1
  LeftShift11/1 -> BitwiseAND11/1
  BitwiseAND11/1 -> [Byte_6_CAN3_CellUnconsistErr]
  bus_selector/13 -> [CAN3_ChrgInLockReq]  "<CAN3_ChrgInLockReq>"
  [CAN3_ChrgInLockReq] -> LeftShift12/1
  LeftShift12/1 -> BitwiseAND12/1
  BitwiseAND12/1 -> [Byte_5_CAN3_ChrgInLockReq]
  bus_selector/14 -> [CAN3_ChrgPlugSta]  "<CAN3_ChrgPlugSta>"
  [CAN3_ChrgPlugSta] -> LeftShift13/1
  LeftShift13/1 -> BitwiseAND13/1
  BitwiseAND13/1 -> [Byte_7_CAN3_ChrgPlugSta]
  bus_selector/15 -> [CAN3_DCChrgSysShockErr]  "<CAN3_DCChrgSysShockErr>"
  [CAN3_DCChrgSysShockErr] -> LeftShift14/1
  LeftShift14/1 -> BitwiseAND14/1
  BitwiseAND14/1 -> [Byte_8_CAN3_DCChrgSysShockErr]
  bus_selector/16 -> [CAN3_DisChrgPlugErr]  "<CAN3_DisChrgPlugErr>"
  [CAN3_DisChrgPlugErr] -> LeftShift15/1
  LeftShift15/1 -> BitwiseAND15/1
  BitwiseAND15/1 -> [Byte_5_CAN3_DisChrgPlugErr]
  bus_selector/17 -> [CAN3_ExtChrgSta]  "<CAN3_ExtChrgSta>"
  [CAN3_ExtChrgSta] -> LeftShift16/1
  LeftShift16/1 -> BitwiseAND16/1
  BitwiseAND16/1 -> [Byte_7_CAN3_ExtChrgSta]
  bus_selector/18 -> [CAN3_HVBCellOvrVoltErr]  "<CAN3_HVBCellOvrVoltErr>"
  [CAN3_HVBCellOvrVoltErr] -> LeftShift17/1
  LeftShift17/1 -> BitwiseAND17/1
  BitwiseAND17/1 -> [Byte_5_CAN3_HVBCellOvrVoltErr]
  bus_selector/19 -> [CAN3_HVBCellOvrVoltWarn]  "<CAN3_HVBCellOvrVoltWarn>"
  [CAN3_HVBCellOvrVoltWarn] -> LeftShift18/1
  LeftShift18/1 -> BitwiseAND18/1
  BitwiseAND18/1 -> [Byte_6_CAN3_HVBCellOvrVoltWarn]
  bus_selector/20 -> [CAN3_HVBCellUdrVoltWarn]  "<CAN3_HVBCellUdrVoltWarn>"
  [CAN3_HVBCellUdrVoltWarn] -> LeftShift19/1
  LeftShift19/1 -> BitwiseAND19/1
  BitwiseAND19/1 -> [Byte_6_CAN3_HVBCellUdrVoltWarn]
  bus_selector/21 -> [CAN3_HVBCellUnbalanErr]  "<CAN3_HVBCellUnbalanErr>"
  [CAN3_HVBCellUnbalanErr] -> LeftShift20/1
  LeftShift20/1 -> BitwiseAND20/1
  BitwiseAND20/1 -> [Byte_5_CAN3_HVBCellUnbalanErr]
  bus_selector/22 -> [CAN3_HVBCellUndrVoltErr]  "<CAN3_HVBCellUndrVoltErr>"
  [CAN3_HVBCellUndrVoltErr] -> LeftShift21/1
  LeftShift21/1 -> BitwiseAND21/1
  BitwiseAND21/1 -> [Byte_5_CAN3_HVBCellUndrVoltErr]
  bus_selector/23 -> [CAN3_HVBChrgErr]  "<CAN3_HVBChrgErr>"
  [CAN3_HVBChrgErr] -> LeftShift22/1
  LeftShift22/1 -> BitwiseAND22/1
  BitwiseAND22/1 -> [Byte_4_CAN3_HVBChrgErr]
  bus_selector/24 -> [CAN3_HVBContactorSta]  "<CAN3_HVBContactorSta>"
  [CAN3_HVBContactorSta] -> LeftShift23/1
  LeftShift23/1 -> BitwiseAND23/1
  BitwiseAND23/1 -> [Byte_8_CAN3_HVBContactorSta]
  bus_selector/25 -> [CAN3_HVBHVILErr]  "<CAN3_HVBHVILErr>"
  [CAN3_HVBHVILErr] -> LeftShift24/1
  LeftShift24/1 -> BitwiseAND24/1
  BitwiseAND24/1 -> [Byte_9_CAN3_HVBHVILErr]
  bus_selector/26 -> [CAN3_HVBOvrChrgCurrErr]  "<CAN3_HVBOvrChrgCurrErr>"
  [CAN3_HVBOvrChrgCurrErr] -> LeftShift25/1
  LeftShift25/1 -> BitwiseAND25/1
  BitwiseAND25/1 -> [Byte_9_CAN3_HVBOvrChrgCurrErr]
  bus_selector/27 -> [CAN3_HVBOvrDchrgCurErr]  "<CAN3_HVBOvrDchrgCurErr>"
  [CAN3_HVBOvrDchrgCurErr] -> LeftShift26/1
  LeftShift26/1 -> BitwiseAND26/1
  BitwiseAND26/1 -> [Byte_9_CAN3_HVBOvrDchrgCurErr]
  bus_selector/28 -> [CAN3_HVBOvrSOCErr]  "<CAN3_HVBOvrSOCErr>"
  [CAN3_HVBOvrSOCErr] -> LeftShift27/1
  LeftShift27/1 -> BitwiseAND27/1
  BitwiseAND27/1 -> [Byte_9_CAN3_HVBOvrSOCErr]
  bus_selector/29 -> [CAN3_HVBOvrTempErr]  "<CAN3_HVBOvrTempErr>"
  [CAN3_HVBOvrTempErr] -> LeftShift28/1
  LeftShift28/1 -> BitwiseAND28/1
  BitwiseAND28/1 -> [Byte_9_CAN3_HVBOvrTempErr]
  bus_selector/30 -> [CAN3_HVBOvrTempWarn]  "<CAN3_HVBOvrTempWarn>"
  [CAN3_HVBOvrTempWarn] -> LeftShift29/1
  LeftShift29/1 -> BitwiseAND29/1
  BitwiseAND29/1 -> [Byte_10_CAN3_HVBOvrTempWarn]
  bus_selector/31 -> [CAN3_HVBOvrVoltErr]  "<CAN3_HVBOvrVoltErr>"
  [CAN3_HVBOvrVoltErr] -> LeftShift30/1
  LeftShift30/1 -> BitwiseAND30/1
  BitwiseAND30/1 -> [Byte_10_CAN3_HVBOvrVoltErr]
  bus_selector/32 -> [CAN3_HVBPrechrgSta]  "<CAN3_HVBPrechrgSta>"
  [CAN3_HVBPrechrgSta] -> LeftShift31/1
  LeftShift31/1 -> BitwiseAND31/1
  BitwiseAND31/1 -> [Byte_8_CAN3_HVBPrechrgSta]
  bus_selector/33 -> [CAN3_HVBPreheatPrecoolSta]  "<CAN3_HVBPreheatPrecoolSta>"
  [CAN3_HVBPreheatPrecoolSta] -> LeftShift32/1
  LeftShift32/1 -> BitwiseAND32/1
  BitwiseAND32/1 -> [Byte_7_CAN3_HVBPreheatPrecoolSta]
  bus_selector/34 -> [CAN3_HVBSOCJumpError]  "<CAN3_HVBSOCJumpError>"
  [CAN3_HVBSOCJumpError] -> LeftShift33/1
  LeftShift33/1 -> BitwiseAND33/1
  BitwiseAND33/1 -> [Byte_9_CAN3_HVBSOCJumpError]
  bus_selector/35 -> [CAN3_HVBShrtChrgCurrErr]  "<CAN3_HVBShrtChrgCurrErr>"
  [CAN3_HVBShrtChrgCurrErr] -> LeftShift34/1
  LeftShift34/1 -> BitwiseAND34/1
  BitwiseAND34/1 -> [Byte_10_CAN3_HVBShrtChrgCurrErr]
  bus_selector/36 -> [CAN3_HVBShrtDischrgCurrErr]  "<CAN3_HVBShrtDischrgCurrErr>"
  [CAN3_HVBShrtDischrgCurrErr] -> LeftShift35/1
  LeftShift35/1 -> BitwiseAND35/1
  BitwiseAND35/1 -> [Byte_10_CAN3_HVBShrtDischrgCurrErr]
  bus_selector/37 -> [CAN3_HVBTempDiffErr]  "<CAN3_HVBTempDiffErr>"
  [CAN3_HVBTempDiffErr] -> LeftShift36/1
  LeftShift36/1 -> BitwiseAND36/1
  BitwiseAND36/1 -> [Byte_8_CAN3_HVBTempDiffErr]
  bus_selector/38 -> [CAN3_HVBUndrSOCErr]  "<CAN3_HVBUndrSOCErr>"
  [CAN3_HVBUndrSOCErr] -> LeftShift37/1
  LeftShift37/1 -> BitwiseAND37/1
  BitwiseAND37/1 -> [Byte_9_CAN3_HVBUndrSOCErr]
  bus_selector/39 -> [CAN3_HVBUndrTempErr]  "<CAN3_HVBUndrTempErr>"
  [CAN3_HVBUndrTempErr] -> LeftShift38/1
  LeftShift38/1 -> BitwiseAND38/1
  BitwiseAND38/1 -> [Byte_9_CAN3_HVBUndrTempErr]
  bus_selector/40 -> [CAN3_HVBUndrTempWarn]  "<CAN3_HVBUndrTempWarn>"
  [CAN3_HVBUndrTempWarn] -> LeftShift39/1
  LeftShift39/1 -> BitwiseAND39/1
  BitwiseAND39/1 -> [Byte_10_CAN3_HVBUndrTempWarn]
  bus_selector/41 -> [CAN3_HVBUndrVoltErr]  "<CAN3_HVBUndrVoltErr>"
  [CAN3_HVBUndrVoltErr] -> LeftShift40/1
  LeftShift40/1 -> BitwiseAND40/1
  BitwiseAND40/1 -> [Byte_10_CAN3_HVBUndrVoltErr]
  bus_selector/42 -> [CAN3_HVBattReady4Pre]  "<CAN3_HVBattReady4Pre>"
  [CAN3_HVBattReady4Pre] -> LeftShift41/1
  LeftShift41/1 -> BitwiseAND41/1
  BitwiseAND41/1 -> [Byte_7_CAN3_HVBattReady4Pre]
  bus_selector/43 -> [CAN3_HVILSta]  "<CAN3_HVILSta>"
  [CAN3_HVILSta] -> LeftShift42/1
  LeftShift42/1 -> BitwiseAND42/1
  BitwiseAND42/1 -> [Byte_8_CAN3_HVILSta]
  bus_selector/44 -> [CAN3_IsoDetSta]  "<CAN3_IsoDetSta>"
  [CAN3_IsoDetSta] -> LeftShift43/1
  LeftShift43/1 -> BitwiseAND43/1
  BitwiseAND43/1 -> [Byte_6_CAN3_IsoDetSta]
  bus_selector/45 -> [CAN3_SystemUncomErr]  "<CAN3_SystemUncomErr>"
  [CAN3_SystemUncomErr] -> LeftShift44/1
  LeftShift44/1 -> BitwiseAND44/1
  BitwiseAND44/1 -> [Byte_6_CAN3_SystemUncomErr]
  bus_selector/46 -> [CAN3_V2LSta]  "<CAN3_V2LSta>"
  [CAN3_V2LSta] -> LeftShift45/1
  LeftShift45/1 -> BitwiseAND45/1
  BitwiseAND45/1 -> [Byte_3_CAN3_V2LSta]
  Data Type Conversion/1 -> BitwiseOR/1
  [Byte_0_CAN3_BMSChckSum] -> Data Type Conversion/1
  BitwiseOR/1 -> [Byte_0]
  Data Type Conversion1/1 -> BitwiseOR1/1
  [Byte_1_CAN3_BMSRolCnct] -> Data Type Conversion1/1
  BitwiseOR1/1 -> [Byte_1]
  constant/1 -> [Byte_2]
  Data Type Conversion2/1 -> BitwiseOR2/1
  [Byte_3_CAN3_V2LSta] -> Data Type Conversion2/1
  BitwiseOR2/1 -> [Byte_3]
  Data Type Conversion3/1 -> BitwiseOR3/1
  [Byte_4_CAN3_HVBChrgErr] -> Data Type Conversion3/1
  BitwiseOR3/1 -> [Byte_4]
  Data Type Conversion4/1 -> BitwiseOR4/1
  [Byte_5_CAN3_ChrgInLockReq] -> Data Type Conversion4/1
  Data Type Conversion5/1 -> BitwiseOR4/2
  [Byte_5_CAN3_DisChrgPlugErr] -> Data Type Conversion5/1
  Data Type Conversion6/1 -> BitwiseOR4/3
  [Byte_5_CAN3_HVBCellOvrVoltErr] -> Data Type Conversion6/1
  Data Type Conversion7/1 -> BitwiseOR4/4
  [Byte_5_CAN3_HVBCellUnbalanErr] -> Data Type Conversion7/1
  Data Type Conversion8/1 -> BitwiseOR4/5
  [Byte_5_CAN3_HVBCellUndrVoltErr] -> Data Type Conversion8/1
  BitwiseOR4/1 -> [Byte_5]
  Data Type Conversion9/1 -> BitwiseOR5/1
  [Byte_6_CAN3_CellUnconsistErr] -> Data Type Conversion9/1
  Data Type Conversion10/1 -> BitwiseOR5/2
  [Byte_6_CAN3_HVBCellOvrVoltWarn] -> Data Type Conversion10/1
  Data Type Conversion11/1 -> BitwiseOR5/3
  [Byte_6_CAN3_HVBCellUdrVoltWarn] -> Data Type Conversion11/1
  Data Type Conversion12/1 -> BitwiseOR5/4
  [Byte_6_CAN3_IsoDetSta] -> Data Type Conversion12/1
  Data Type Conversion13/1 -> BitwiseOR5/5
  [Byte_6_CAN3_SystemUncomErr] -> Data Type Conversion13/1
  BitwiseOR5/1 -> [Byte_6]
  Data Type Conversion14/1 -> BitwiseOR6/1
  [Byte_7_CAN3_ChrgPlugSta] -> Data Type Conversion14/1
  Data Type Conversion15/1 -> BitwiseOR6/2
  [Byte_7_CAN3_ExtChrgSta] -> Data Type Conversion15/1
  Data Type Conversion16/1 -> BitwiseOR6/3
  [Byte_7_CAN3_HVBPreheatPrecoolSta] -> Data Type Conversion16/1
  Data Type Conversion17/1 -> BitwiseOR6/4
  [Byte_7_CAN3_HVBattReady4Pre] -> Data Type Conversion17/1
  BitwiseOR6/1 -> [Byte_7]
  Data Type Conversion18/1 -> BitwiseOR7/1
  [Byte_8_CAN3_BMS_READY] -> Data Type Conversion18/1
  Data Type Conversion19/1 -> BitwiseOR7/2
  [Byte_8_CAN3_DCChrgSysShockErr] -> Data Type Conversion19/1
  Data Type Conversion20/1 -> BitwiseOR7/3
  [Byte_8_CAN3_HVBContactorSta] -> Data Type Conversion20/1
  Data Type Conversion21/1 -> BitwiseOR7/4
  [Byte_8_CAN3_HVBPrechrgSta] -> Data Type Conversion21/1
  Data Type Conversion22/1 -> BitwiseOR7/5
  [Byte_8_CAN3_HVBTempDiffErr] -> Data Type Conversion22/1
  Data Type Conversion23/1 -> BitwiseOR7/6
  [Byte_8_CAN3_HVILSta] -> Data Type Conversion23/1
  BitwiseOR7/1 -> [Byte_8]
  Data Type Conversion24/1 -> BitwiseOR8/1
  [Byte_9_CAN3_HVBHVILErr] -> Data Type Conversion24/1
  Data Type Conversion25/1 -> BitwiseOR8/2
  [Byte_9_CAN3_HVBOvrChrgCurrErr] -> Data Type Conversion25/1
  Data Type Conversion26/1 -> BitwiseOR8/3
  [Byte_9_CAN3_HVBOvrDchrgCurErr] -> Data Type Conversion26/1
  Data Type Conversion27/1 -> BitwiseOR8/4
  [Byte_9_CAN3_HVBOvrSOCErr] -> Data Type Conversion27/1
  Data Type Conversion28/1 -> BitwiseOR8/5
  [Byte_9_CAN3_HVBOvrTempErr] -> Data Type Conversion28/1
  Data Type Conversion29/1 -> BitwiseOR8/6
  [Byte_9_CAN3_HVBSOCJumpError] -> Data Type Conversion29/1
  Data Type Conversion30/1 -> BitwiseOR8/7
  [Byte_9_CAN3_HVBUndrSOCErr] -> Data Type Conversion30/1
  Data Type Conversion31/1 -> BitwiseOR8/8
  [Byte_9_CAN3_HVBUndrTempErr] -> Data Type Conversion31/1
  BitwiseOR8/1 -> [Byte_9]
  Data Type Conversion32/1 -> BitwiseOR9/1
  [Byte_10_CAN3_HVBOvrTempWarn] -> Data Type Conversion32/1
  Data Type Conversion33/1 -> BitwiseOR9/2
  [Byte_10_CAN3_HVBOvrVoltErr] -> Data Type Conversion33/1
  Data Type Conversion34/1 -> BitwiseOR9/3
  [Byte_10_CAN3_HVBShrtChrgCurrErr] -> Data Type Conversion34/1
  Data Type Conversion35/1 -> BitwiseOR9/4
  [Byte_10_CAN3_HVBShrtDischrgCurrErr] -> Data Type Conversion35/1
  Data Type Conversion36/1 -> BitwiseOR9/5
  [Byte_10_CAN3_HVBUndrTempWarn] -> Data Type Conversion36/1
  Data Type Conversion37/1 -> BitwiseOR9/6
  [Byte_10_CAN3_HVBUndrVoltErr] -> Data Type Conversion37/1
  BitwiseOR9/1 -> [Byte_10]
  Data Type Conversion38/1 -> BitwiseOR10/1
  [Byte_11_CAN3_BMS_Warn_1] -> Data Type Conversion38/1
  Data Type Conversion39/1 -> BitwiseOR10/2
  [Byte_11_CAN3_BMS_Warn_2] -> Data Type Conversion39/1
  Data Type Conversion40/1 -> BitwiseOR10/3
  [Byte_11_CAN3_BMS_Warn_3] -> Data Type Conversion40/1
  Data Type Conversion41/1 -> BitwiseOR10/4
  [Byte_11_CAN3_BMS_Warn_4] -> Data Type Conversion41/1
  Data Type Conversion42/1 -> BitwiseOR10/5
  [Byte_11_CAN3_BMS_Warn_5] -> Data Type Conversion42/1
  Data Type Conversion43/1 -> BitwiseOR10/6
  [Byte_11_CAN3_BMS_Warn_6] -> Data Type Conversion43/1
  Data Type Conversion44/1 -> BitwiseOR10/7
  [Byte_11_CAN3_BMS_Warn_7] -> Data Type Conversion44/1
  Data Type Conversion45/1 -> BitwiseOR10/8
  [Byte_11_CAN3_BMS_Warn_8] -> Data Type Conversion45/1
  BitwiseOR10/1 -> [Byte_11]
  [Byte_1] -> Mux/1
  [Byte_2] -> Mux/2
  [Byte_3] -> Mux/3
  [Byte_4] -> Mux/4
  [Byte_5] -> Mux/5
  [Byte_6] -> Mux/6
  [Byte_7] -> Mux/7
  [Byte_8] -> Mux/8
  [Byte_9] -> Mux/9
  [Byte_10] -> Mux/10
  [Byte_11] -> Mux/11
  Mux/1 -> [VHAL_CAN3BMS6noCS_raw]
  KHAL_CAN3BMS6E2E_flg/1 -> DDM_CS&RC_Comparison/1
  0x3B/1 -> DDM_CS&RC_Comparison/2
  0xDB/1 -> DDM_CS&RC_Comparison/3
  [VHAL_CAN3BMS6noCS_raw] -> DDM_CS&RC_Comparison/4
  [Byte_0] -> DDM_CS&RC_Comparison/5
  [RC_ECU] -> DDM_CS&RC_Comparison/6
  MessageRollingCounter/1 -> DDM_CS&RC_Comparison/7
  DDM_CS&RC_Comparison/1 -> VHAL_BMS6CSErr_flg/1
  DDM_CS&RC_Comparison/2 -> VHAL_BMS6RCErr_flg/1
  [DT_CAN3_SG_BMS6] -> bus_selector1/1
  bus_selector1/1 -> BMSChckSum/1(BMSChckSum)  "<CAN3_BMSChckSum>"
  BMSChckSum/1(VHAL_BMSChckSum_enum) -> VHAL_BMSChckSum_enum/1
  [DT_CAN3_SG_BMS6] -> bus_selector2/1
  bus_selector2/1 -> BMSRolCnct/1(BMSRolCnct)  "<CAN3_BMSRolCnct>"
  BMSRolCnct/1(VHAL_BMSRolCnct_enum) -> VHAL_BMSRolCnct_enum/1, [RC_ECU]
  [DT_CAN3_SG_BMS6] -> bus_selector3/1
  bus_selector3/1 -> BMSREADY/1(BMS_READY)  "<CAN3_BMS_READY>"
  BMSREADY/1(VHAL_BMSREADY_flg) -> VHAL_BMSREADY_flg/1
  [DT_CAN3_SG_BMS6] -> bus_selector4/1
  bus_selector4/1 -> BMSWarn1/1(BMS_Warn_1)  "<CAN3_BMS_Warn_1>"
  BMSWarn1/1(VHAL_BMSWarn1_flg) -> VHAL_BMSWarn1_flg/1
  [DT_CAN3_SG_BMS6] -> bus_selector5/1
  bus_selector5/1 -> BMSWarn2/1(BMS_Warn_2)  "<CAN3_BMS_Warn_2>"
  BMSWarn2/1(VHAL_BMSWarn2_flg) -> VHAL_BMSWarn2_flg/1
  [DT_CAN3_SG_BMS6] -> bus_selector6/1
  bus_selector6/1 -> BMSWarn3/1(BMS_Warn_3)  "<CAN3_BMS_Warn_3>"
  BMSWarn3/1(VHAL_BMSWarn3_flg) -> VHAL_BMSWarn3_flg/1
  [DT_CAN3_SG_BMS6] -> bus_selector7/1
  bus_selector7/1 -> BMSWarn4/1(BMS_Warn_4)  "<CAN3_BMS_Warn_4>"
  BMSWarn4/1(VHAL_BMSWarn4_flg) -> VHAL_BMSWarn4_flg/1
  [DT_CAN3_SG_BMS6] -> bus_selector8/1
  bus_selector8/1 -> BMSWarn5/1(BMS_Warn_5)  "<CAN3_BMS_Warn_5>"
  BMSWarn5/1(VHAL_BMSWarn5_flg) -> VHAL_BMSWarn5_flg/1
  [DT_CAN3_SG_BMS6] -> bus_selector9/1
  bus_selector9/1 -> BMSWarn6/1(BMS_Warn_6)  "<CAN3_BMS_Warn_6>"
  BMSWarn6/1(VHAL_BMSWarn6_flg) -> VHAL_BMSWarn6_flg/1
  [DT_CAN3_SG_BMS6] -> bus_selector10/1
  bus_selector10/1 -> BMSWarn7/1(BMS_Warn_7)  "<CAN3_BMS_Warn_7>"
  BMSWarn7/1(VHAL_BMSWarn7_flg) -> VHAL_BMSWarn7_flg/1
  [DT_CAN3_SG_BMS6] -> bus_selector11/1
  bus_selector11/1 -> BMSWarn8/1(BMS_Warn_8)  "<CAN3_BMS_Warn_8>"
  BMSWarn8/1(VHAL_BMSWarn8_flg) -> VHAL_BMSWarn8_flg/1
  [DT_CAN3_SG_BMS6] -> bus_selector12/1
  bus_selector12/1 -> ChrgInLockReq/1(ChrgInLockReq)  "<CAN3_ChrgInLockReq>"
  ChrgInLockReq/1(VHAL_ChrgInLockReq_enum) -> VHAL_ChrgInLockReq_enum/1
  [DT_CAN3_SG_BMS6] -> bus_selector13/1
  bus_selector13/1 -> ChrgPlugSta/1(ChrgPlugSta)  "<CAN3_ChrgPlugSta>"
  ChrgPlugSta/1(VHAL_ChrgPlugSta_enum) -> VHAL_ChrgPlugSta_enum/1
  [DT_CAN3_SG_BMS6] -> bus_selector14/1
  bus_selector14/1 -> DisChrgPlugErr/1(DisChrgPlugErr)  "<CAN3_DisChrgPlugErr>"
  DisChrgPlugErr/1(VHAL_DisChrgPlugErr_enum) -> VHAL_DisChrgPlugErr_enum/1
  [DT_CAN3_SG_BMS6] -> bus_selector15/1
  bus_selector15/1 -> ExtChrgSta/1(ExtChrgSta)  "<CAN3_ExtChrgSta>"
  ExtChrgSta/1(VHAL_ExtChrgSta_enum) -> VHAL_ExtChrgSta_enum/1
  [DT_CAN3_SG_BMS6] -> bus_selector16/1
  bus_selector16/1 -> HVBChrgErr/1(HVBChrgErr)  "<CAN3_HVBChrgErr>"
  HVBChrgErr/1(VHAL_HVBChrgErr_enum) -> VHAL_HVBChrgErr_enum/1
  [DT_CAN3_SG_BMS6] -> bus_selector17/1
  bus_selector17/1 -> HVBContactorSta/1(HVBContactorSta)  "<CAN3_HVBContactorSta>"
  HVBContactorSta/1(VHAL_HVBContactorSta_flg) -> VHAL_HVBContactorSta_flg/1
  [DT_CAN3_SG_BMS6] -> bus_selector18/1
  bus_selector18/1 -> HVBHVILErr/1(HVBHVILErr)  "<CAN3_HVBHVILErr>"
  HVBHVILErr/1(VHAL_HVBHVILErr_flg) -> VHAL_HVBHVILErr_flg/1
  [DT_CAN3_SG_BMS6] -> bus_selector19/1
  bus_selector19/1 -> HVBOvrTempErr/1(HVBOvrTempErr)  "<CAN3_HVBOvrTempErr>"
  HVBOvrTempErr/1(VHAL_HVBOvrTempErr_flg) -> VHAL_HVBOvrTempErr_flg/1
  [DT_CAN3_SG_BMS6] -> bus_selector20/1
  bus_selector20/1 -> HVBOvrTempWarn/1(HVBOvrTempWarn)  "<CAN3_HVBOvrTempWarn>"
  HVBOvrTempWarn/1(VHAL_HVBOvrTempWarn_enum) -> VHAL_HVBOvrTempWarn_enum/1
  [DT_CAN3_SG_BMS6] -> bus_selector21/1
  bus_selector21/1 -> HVBPreheatPrecoolSta/1(HVBPreheatPrecoolSta)  "<CAN3_HVBPreheatPrecoolSta>"
  HVBPreheatPrecoolSta/1(VHAL_HVBPreheatPrecoolSta_enum) -> VHAL_HVBPreheatPrecoolSta_enum/1
  [DT_CAN3_SG_BMS6] -> bus_selector22/1
  bus_selector22/1 -> HVBattReady4Pre/1(HVBattReady4Pre)  "<CAN3_HVBattReady4Pre>"
  HVBattReady4Pre/1(VHAL_HVBattReady4Pre_enum) -> VHAL_HVBattReady4Pre_enum/1
  [DT_CAN3_SG_BMS6] -> bus_selector23/1
  bus_selector23/1 -> HVILSta/1(HVILSta)  "<CAN3_HVILSta>"
  HVILSta/1(VHAL_HVILSta_flg) -> VHAL_HVILSta_flg/1
  [DT_CAN3_SG_BMS6] -> bus_selector24/1
  bus_selector24/1 -> V2LSta/1(V2LSta)  "<CAN3_V2LSta>"
  V2LSta/1(VHAL_V2LSta_enum) -> VHAL_V2LSta_enum/1

== system halin/HAL_IN/CAN3/BMS8 ==
  DT_CAN3_SG_BMS8 : Inport
  MainRlyNegSta : Subsystem
  MainRlyPosSta : Subsystem
  bus_selector : BusSelector  OutputSignals=CAN3_MainRlyNegSta
  bus_selector1 : BusSelector  OutputSignals=CAN3_MainRlyPosSta
  VHAL_MainRlyNegSta_enum : Outport
  VHAL_MainRlyPosSta_enum : Outport  Port=2
  wires:
  DT_CAN3_SG_BMS8/1 -> [DT_CAN3_SG_BMS8]
  [DT_CAN3_SG_BMS8] -> bus_selector/1
  bus_selector/1 -> MainRlyNegSta/1(MainRlyNegSta)  "<CAN3_MainRlyNegSta>"
  MainRlyNegSta/1(VHAL_MainRlyNegSta_enum) -> VHAL_MainRlyNegSta_enum/1
  [DT_CAN3_SG_BMS8] -> bus_selector1/1
  bus_selector1/1 -> MainRlyPosSta/1(MainRlyPosSta)  "<CAN3_MainRlyPosSta>"
  MainRlyPosSta/1(VHAL_MainRlyPosSta_enum) -> VHAL_MainRlyPosSta_enum/1
